simulink model "AMCLIB_FW_BAM"  (Simulink 9.3)
settings: Solver=VariableStepAuto  StartTime=0.0  StopTime=10.0  RelTol=1e-3
settings Model: Creator=nxa18952  LastModifiedBy=nxa18952
settings DataIOCC: SaveFormat=Dataset  SignalLoggingSaveFormat=Dataset  ReturnWorkspaceOutputs=on
settings OptimizationCC: LifeSpan=auto
settings DebuggingCC: UnderspecifiedInitializationDetection=Simplified  MergeDetectMultiDrivingBlocksExec=error  FcnCallInpInsideContextMsg=error  SFUnexpectedBacktrackingDiag=error  SFNoUnconditionalDefaultTransitionDiag=error  SFExecutionAtInitializationDiag=warning  ArithmeticOperatorsInVariantConditions=error
settings HardwareCC: ProdBitPerPointer=64  ProdBitPerSizeT=64  ProdBitPerPtrDiffT=64  ProdLargestAtomicFloat=Float  ProdIntDivRoundTo=Zero  ProdEndianess=LittleEndian  ProdWordSize=64  ProdHWDeviceType=Intel->x86-64 (Windows64)
settings ModelReferenceCC: PropagateSignalLabelsOutOfModel=on
settings SFSimCC: SimUseLocalCustomCode=on
settings RTWCC: RTWUseLocalCustomCode=on
settings CodeAppCC: StateflowObjectComments=off
settings GRTTargetCC: TargetLangStandard=C99 (ISO)  CombineOutputUpdateFcns=on  GRTInterface=off
settings ConfigComp: CovMetricSettings=dwe  CovHtmlReporting=off  CovSaveCumulativeToWorkspaceVar=off  CovSaveSingleToWorkspaceVar=off  CovExternalEMLEnable=on

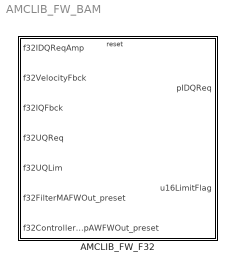
== system AMCLIB_FW_BAM ==
  AMCLIB_FW_F32 : Subsystem  TreatAsAtomicUnit=on  mask(AMCLIB_FW_F32){showStates=Hide (faster execution), resetStatesEnable=Pre-set according to the first set of inputs after reset, showDebugOutputs=Hide, u16NSamples=0, f32PropGain=0, f32IntegGain=0, s16PropGainShift=0, s16IntegGainShift=0, f32LowerLimit=0, f32UpperLimit=0}
      mask prompts: showStates "Show internal states"; resetStatesEnable "Internal state after reset"; showDebugOutputs "Show debugging outputs"; u16NSamples "u16NSamples (GDFLIB_FilterMA - recalculated smoothing factor)"; f32PropGain "f32PropGain (GFLIB_ControllerPIpAW - proportional gain)"; f32IntegGain "f32IntegGain (GFLIB_ControllerPIpAW - integral gain)"; s16PropGainShift "s16PropGainShift (GFLIB_ControllerPIpAW - scaling bitwise shift applied to the proportional gain)"; s16IntegGainShift "s16IntegGainShift (GFLIB_ControllerPIpAW - scaling bitwise shift applied to the integral gain)"; f32LowerLimit "f32LowerLimit (GFLIB_ControllerPIpAW - lower limit)"; f32UpperLimit "f32UpperLimit (GFLIB_ControllerPIpAW - upper limit)"
      mask help: Field Weakening controller for the PMSM field-oriented control algorithm in 32-bit fixed-point fractional implementation. This block supports re-initialization of the internal state during simulation. If the block is reset, the output of the MA filter and PI controller will be aligned with the inputs f32FilterMAFWOut_preset and f32ControllerPIpAWFWOut_preset. Refer to the AMMCLIB User's Guide for further details.
      mask init:
      | if ~evalin('base','exist(''tS8'',''var'')')
      |   if (2 ~= exist('SWLIBS_Typedefs.mat','file'))
      |       error('File SWLIBS_Typedefs.mat is not on the Matlab path. Please add the AMMCLIB "bam" folder in the Matlab Search Path.');
      |   else
      |       evalin('base', 'load(''SWLIBS_Typedefs.mat'')');
      |   end
      | end
      | if showStates == 1
      |     % hidden state variables
      |     if strcmp(get_param([gcb '/u16NSamples'], 'BlockType'), 'Inport')
      |         posblk = get_param(gcb, 'Position');
      | 
      |         pos = get_param(    [gcb, '/u16NSamples'], 'Position');
      |         orient = get_param( [gcb, '/u16NSamples'], 'Orientation');
      |         delete_block(       [gcb, '/u16NSamples']);
      |         add_block('built-in/Ground', [gcb, '/u16NSamples'], 'Position', pos, 'Orientation', orient);
      | 
      |         pos = get_param(    [gcb, '/f32PropGain'], 'Position');
      |         orient = get_param( [gcb, '/f32PropGain'], 'Orientation');
      |         delete_block(       [gcb, '/f32PropGain']);
      |         add_block('built-in/Ground', [gcb, '/f32PropGain'], 'Position', pos, 'Orientation', orient);
      | 
      |         pos = get_param(    [gcb, '/f32IntegGain'], 'Position');
      |         orient = get_param( [gcb, '/f32IntegGain'], 'Orientation');
      |         delete_block(       [gcb, '/f32IntegGain']);
      |         add_block('built-in/Ground', [gcb, '/f32IntegGain'], 'Position', pos, 'Orientation', orient);
      | 
      |         pos = get_param(    [gcb, '/s16PropGainShift'], 'Position');
      |         orient = get_param( [gcb, '/s16PropGainShift'], 'Orientation');
      |         delete_block(       [gcb, '/s16PropGainShift']);
      |         add_block('built-in/Ground', [gcb, '/s16PropGainShift'], 'Position', pos, 'Orientation', orient);
      | 
      |         pos = get_param(    [gcb, '/s16IntegGainShift'], 'Position');
      |         orient = get_param( [gcb, '/s16IntegGainShift'], 'Orientation');
      |         delete_block(       [gcb, '/s16IntegGainShift']);
      |         add_block('built-in/Ground', [gcb, '/s16IntegGainShift'], 'Position', pos, 'Orientation', orient);
      | 
      |         pos = get_param(    [gcb, '/f32LowerLimit'], 'Position');
      |         orient = get_param( [gcb, '/f32LowerLimit'], 'Orientation');
      |         delete_block(       [gcb, '/f32LowerLimit']);
      |         add_block('built-in/Ground', [gcb, '/f32LowerLimit'], 'Position', pos, 'Orientation', orient);
      | 
      |         pos = get_param(    [gcb, '/f32UpperLimit'], 'Position');
      |         orient = get_param( [gcb, '/f32UpperLimit'], 'Orientation');
      |         delete_block(       [gcb, '/f32UpperLimit']);
      |         add_block('built-in/Ground', [gcb, '/f32UpperLimit'], 'Position', pos, 'Orientation', orient);
      | 
      |         pos = get_param(    [gcb, '/f32IQReqK_1'], 'Position');
      |         orient = get_param( [gcb, '/f32IQReqK_1'], 'Orientation');
      |         delete_block(       [gcb, '/f32IQReqK_1']);
      |         add_block('built-in/Ground', [gcb, '/f32IQReqK_1'], 'Position', pos, 'Orientation', orient);
      | 
      |         pos = get_param(    [gcb, '/f32Acc'], 'Position');
      |         orient = get_param( [gcb, '/f32Acc'], 'Orientation');
      |         delete_block(       [gcb, '/f32Acc']);
      |         add_block('built-in/Ground', [gcb, '/f32Acc'], 'Position', pos, 'Orientation', orient);
      | 
      |         pos = get_param(    [gcb, '/f32IntegPartK_1'], 'Position');
      |         orient = get_param( [gcb, '/f32IntegPartK_1'], 'Orientation');
      |         delete_block(       [gcb, '/f32IntegPartK_1']);
      |         add_block('built-in/Ground', [gcb, '/f32IntegPartK_1'], 'Position', pos, 'Orientation', orient);
      | 
      |         pos = get_param(    [gcb, '/f32InK_1'], 'Position');
      |         orient = get_param( [gcb, '/f32InK_1'], 'Orientation');
      |         delete_block(       [gcb, '/f32InK_1']);
      |         add_block('built-in/Ground', [gcb, '/f32InK_1'], 'Position', pos, 'Orientation', orient);
      | 
      | 
      |         pos = get_param(    [gcb '/f32Acc_Out'], 'Position');
      |         orient = get_param( [gcb '/f32Acc_Out'], 'Orientation');
      |         delete_block(       [gcb '/f32Acc_Out']);
      |         add_block('built-in/Terminator', [gcb '/f32Acc_Out'], 'Position', pos, 'Orientation', orient);
      | 
      |         pos = get_param(    [gcb '/f32IntegPartK_1_Out'], 'Position');
      |         orient = get_param( [gcb '/f32IntegPartK_1_Out'], 'Orientation');
      |         delete_block(       [gcb '/f32IntegPartK_1_Out']);
      |         add_block('built-in/Terminator', [gcb '/f32IntegPartK_1_Out'], 'Position', pos, 'Orientation', orient);
      | 
      |         pos = get_param(    [gcb '/f32InK_1_Out'], 'Position');
      |         orient = get_param( [gcb '/f32InK_1_Out'], 'Orientation');
      |         delete_block(       [gcb '/f32InK_1_Out']);
      |         add_block('built-in/Terminator', [gcb '/f32InK_1_Out'], 'Position', pos, 'Orientation', orient);
      | 
      | 
      |         if strcmp(get_param([gcb '/f32IQErrSign'], 'BlockType'), 'Outport')
      |             pos = get_param(    [gcb '/f32IQErrSign'], 'Position');
      |             orient = get_param( [gcb '/f32IQErrSign'], 'Orientation');
      |             delete_block(       [gcb '/f32IQErrSign']);
      |             add_block('built-in/Terminator', [gcb '/f32IQErrSign'], 'Position', pos, 'Orientation', orient);
      | 
      |             pos = get_param(    [gcb '/f32IQErr'], 'Position');
      |             orient = get_param( [gcb '/f32IQErr'], 'Orientation');
      |             delete_block(       [gcb '/f32IQErr']);
      |             add_block('built-in/Terminator', [gcb '/f32IQErr'], 'Position', pos, 'Orientation', orient);
      | 
      |             pos = get_param(    [gcb '/f32FWErr'], 'Position');
      |             orient = get_param( [gcb '/f32FWErr'], 'Orientation');
      |             delete_block(       [gcb '/f32FWErr']);
      |             add_block('built-in/Terminator', [gcb '/f32FWErr'], 'Position', pos, 'Orientation', orient);
      | 
      |             pos = get_param(    [gcb '/f32UQErr'], 'Position');
      |             orient = get_param( [gcb '/f32UQErr'], 'Orientation');
      |             delete_block(       [gcb '/f32UQErr']);
      |             add_block('built-in/Terminator', [gcb '/f32UQErr'], 'Position', pos, 'Orientation', orient);
      | 
      |             pos = get_param(    [gcb '/f32FWErrFilt'], 'Position');
      |             orient = get_param( [gcb '/f32FWErrFilt'], 'Orientation');
      |             delete_block(       [gcb '/f32FWErrFilt']);
      |             add_block('built-in/Terminator', [gcb '/f32FWErrFilt'], 'Position', pos, 'Orientation', orient);
      | 
      |             pos = get_param(    [gcb '/f32FWAngle'], 'Position');
      |             orient = get_param( [gcb '/f32FWAngle'], 'Orientation');
      |             delete_block(       [gcb '/f32FWAngle']);
      |             add_block('built-in/Terminator', [gcb '/f32FWAngle'], 'Position', pos, 'Orientation', orient);
      | 
      |             pos = get_param(    [gcb '/f32FWSin'], 'Position');
      |             orient = get_param( [gcb '/f32FWSin'], 'Orientation');
      |             delete_block(       [gcb '/f32FWSin']);
      |             add_block('built-in/Terminator', [gcb '/f32FWSin'], 'Position', pos, 'Orientation', orient);
      | 
      |             pos = get_param(    [gcb '/f32FWCos'], 'Position');
      |             orient = get_param( [gcb '/f32FWCos'], 'Orientation');
      |             delete_block(       [gcb '/f32FWCos']);
      |             add_block('built-in/Terminator', [gcb '/f32FWCos'], 'Position', pos, 'Orientation', orient);
      | 
      |         end
      | 
      |         set_param([gcb '/f32IDQReqAmp'], 'Port', '1');
      |         set_param([gcb '/f32VelocityFbck'], 'Port', '2');
      |         set_param([gcb '/f32IQFbck'], 'Port', '3');
      |         set_param([gcb '/f32UQReq'], 'Port', '4');
      |         set_param([gcb '/f32UQLim'], 'Port', '5');
      |         set_param([gcb '/f32FilterMAFWOut_preset'], 'Port', '6');
      |         set_param([gcb '/f32ControllerPIpAWFWOut_preset'], 'Port', '7');
      | 
      |         set_param([gcb '/pIDQReq'], 'Port', '1');
      |         set_param([gcb '/u16LimitFlag'], 'Port', '2');
      | 
      |         set_param(gcb,'MaskEnables',{'on','on','off','on','on','on','on','on','on','on'});
      | 
      |         if (posblk(4) - posblk(2)) > 200
      |           height = 200;
      |           set_param(gcb,'Position',[posblk(1), posblk(2), posblk(3), posblk(2)+height])
      |         end
      |     end
      | else
      |     % shown state variables
      |     if strcmp(get_param([gcb '/u16NSamples'], 'BlockType'), 'Ground')
      |         posblk = get_param(gcb, 'Position');
      | 
      |         pos = get_param(    [gcb, '/u16NSamples'], 'Position');
      |         orient = get_param( [gcb, '/u16NSamples'], 'Orientation');
      |         delete_block(       [gcb, '/u16NSamples']);
      |         add_block('built-in/Inport', [gcb, '/u16NSamples'], 'Position', pos, 'Orientation', orient, 'OutDataTypeStr', 'uint16');
      | 
      |         pos = get_param(    [gcb, '/f32PropGain'], 'Position');
      |         orient = get_param( [gcb, '/f32PropGain'], 'Orientation');
      |         delete_block(       [gcb, '/f32PropGain']);
      |         add_block('built-in/Inport', [gcb, '/f32PropGain'], 'Position', pos, 'Orientation', orient, 'OutDataTypeStr', 'int32');
      | 
      |         pos = get_param(    [gcb, '/f32IntegGain'], 'Position');
      |         orient = get_param( [gcb, '/f32IntegGain'], 'Orientation');
      |         delete_block(       [gcb, '/f32IntegGain']);
      |         add_block('built-in/Inport', [gcb, '/f32IntegGain'], 'Position', pos, 'Orientation', orient, 'OutDataTypeStr', 'int32');
      | 
      |         pos = get_param(    [gcb, '/s16PropGainShift'], 'Position');
      |         orient = get_param( [gcb, '/s16PropGainShift'], 'Orientation');
      |         delete_block(       [gcb, '/s16PropGainShift']);
      |         add_block('built-in/Inport', [gcb, '/s16PropGainShift'], 'Position', pos, 'Orientation', orient, 'OutDataTypeStr', 'int16');
      | 
      |         pos = get_param(    [gcb, '/s16IntegGainShift'], 'Position');
      |         orient = get_param( [gcb, '/s16IntegGainShift'], 'Orientation');
      |         delete_block(       [gcb, '/s16IntegGainShift']);
      |         add_block('built-in/Inport', [gcb, '/s16IntegGainShift'], 'Position', pos, 'Orientation', orient, 'OutDataTypeStr', 'int16');
      | 
      |         pos = get_param(    [gcb, '/f32LowerLimit'], 'Position');
      |         orient = get_param( [gcb, '/f32LowerLimit'], 'Orientation');
      |         delete_block(       [gcb, '/f32LowerLimit']);
      |         add_block('built-in/Inport', [gcb, '/f32LowerLimit'], 'Position', pos, 'Orientation', orient, 'OutDataTypeStr', 'int32');
      | 
      |         pos = get_param(    [gcb, '/f32UpperLimit'], 'Position');
      |         orient = get_param( [gcb, '/f32UpperLimit'], 'Orientation');
      |         delete_block(       [gcb, '/f32UpperLimit']);
      |         add_block('built-in/Inport', [gcb, '/f32UpperLimit'], 'Position', pos, 'Orientation', orient, 'OutDataTypeStr', 'int32');
      | 
      |         pos = get_param(    [gcb, '/f32IQReqK_1'], 'Position');
      |         orient = get_param( [gcb, '/f32IQReqK_1'], 'Orientation');
      |         delete_block(       [gcb, '/f32IQReqK_1']);
      |         add_block('built-in/Inport', [gcb, '/f32IQReqK_1'], 'Position', pos, 'Orientation', orient, 'OutDataTypeStr', 'int32');
      | 
      |         pos = get_param(    [gcb, '/f32Acc'], 'Position');
      |         orient = get_param( [gcb, '/f32Acc'], 'Orientation');
      |         delete_block(       [gcb, '/f32Acc']);
      |         add_block('built-in/Inport', [gcb, '/f32Acc'], 'Position', pos, 'Orientation', orient, 'OutDataTypeStr', 'int32');
      | 
      |         pos = get_param(    [gcb, '/f32IntegPartK_1'], 'Position');
      |         orient = get_param( [gcb, '/f32IntegPartK_1'], 'Orientation');
      |         delete_block(       [gcb, '/f32IntegPartK_1']);
      |         add_block('built-in/Inport', [gcb, '/f32IntegPartK_1'], 'Position', pos, 'Orientation', orient, 'OutDataTypeStr', 'int32');
      | 
      |         pos = get_param(    [gcb, '/f32InK_1'], 'Position');
      |         orient = get_param( [gcb, '/f32InK_1'], 'Orientation');
      |         delete_block(       [gcb, '/f32InK_1']);
      |         add_block('built-in/Inport', [gcb, '/f32InK_1'], 'Position', pos, 'Orientation', orient, 'OutDataTypeStr', 'int32');
      | 
      | 
      |         pos = get_param(    [gcb '/f32Acc_Out'], 'Position');
      |         orient = get_param( [gcb '/f32Acc_Out'], 'Orientation');
      |         delete_block(       [gcb '/f32Acc_Out']);
      |         add_block('built-in/Outport', [gcb '/f32Acc_Out'], 'Position', pos, 'Orientation', orient);
      | 
      |         pos = get_param(    [gcb '/f32IntegPartK_1_Out'], 'Position');
      |         orient = get_param( [gcb '/f32IntegPartK_1_Out'], 'Orientation');
      |         delete_block(       [gcb '/f32IntegPartK_1_Out']);
      |         add_block('built-in/Outport', [gcb '/f32IntegPartK_1_Out'], 'Position', pos, 'Orientation', orient);
      | 
      |         pos = get_param(    [gcb '/f32InK_1_Out'], 'Position');
      |         orient = get_param( [gcb '/f32InK_1_Out'], 'Orientation');
      |         delete_block(       [gcb '/f32InK_1_Out']);
      |         add_block('built-in/Outport', [gcb '/f32InK_1_Out'], 'Position', pos, 'Orientation', orient);
      | 
      | 
      |         if (showDebugOutputs == 2) && (strcmp(get_param([gcb '/f32IQErrSign'], 'BlockType'), 'Terminator'))
      |             pos = get_param(    [gcb '/f32IQErrSign'], 'Position');
      |             orient = get_param( [gcb '/f32IQErrSign'], 'Orientation');
      |             delete_block(       [gcb '/f32IQErrSign']);
      |             add_block('built-in/Outport', [gcb '/f32IQErrSign'], 'Position', pos, 'Orientation', orient);
      | 
      |             pos = get_param(    [gcb '/f32IQErr'], 'Position');
      |             orient = get_param( [gcb '/f32IQErr'], 'Orientation');
      |             delete_block(       [gcb '/f32IQErr']);
      |             add_block('built-in/Outport', [gcb '/f32IQErr'], 'Position', pos, 'Orientation', orient);
      | 
      |             pos = get_param(    [gcb '/f32FWErr'], 'Position');
      |             orient = get_param( [gcb '/f32FWErr'], 'Orientation');
      |             delete_block(       [gcb '/f32FWErr']);
      |             add_block('built-in/Outport', [gcb '/f32FWErr'], 'Position', pos, 'Orientation', orient);
      | 
      |             pos = get_param(    [gcb '/f32UQErr'], 'Position');
      |             orient = get_param( [gcb '/f32UQErr'], 'Orientation');
      |             delete_block(       [gcb '/f32UQErr']);
      |             add_block('built-in/Outport', [gcb '/f32UQErr'], 'Position', pos, 'Orientation', orient);
      | 
      |             pos = get_param(    [gcb '/f32FWErrFilt'], 'Position');
      |             orient = get_param( [gcb '/f32FWErrFilt'], 'Orientation');
      |             delete_block(       [gcb '/f32FWErrFilt']);
      |             add_block('built-in/Outport', [gcb '/f32FWErrFilt'], 'Position', pos, 'Orientation', orient);
      | 
      |             pos = get_param(    [gcb '/f32FWAngle'], 'Position');
      |             orient = get_param( [gcb '/f32FWAngle'], 'Orientation');
      |             delete_block(       [gcb '/f32FWAngle']);
      |             add_block('built-in/Outport', [gcb '/f32FWAngle'], 'Position', pos, 'Orientation', orient);
      | 
      |             pos = get_param(    [gcb '/f32FWSin'], 'Position');
      |             orient = get_param( [gcb '/f32FWSin'], 'Orientation');
      |             delete_block(       [gcb '/f32FWSin']);
      |             add_block('built-in/Outport', [gcb '/f32FWSin'], 'Position', pos, 'Orientation', orient);
      | 
      |             pos = get_param(    [gcb '/f32FWCos'], 'Position');
      |             orient = get_param( [gcb '/f32FWCos'], 'Orientation');
      |             delete_block(       [gcb '/f32FWCos']);
      |             add_block('built-in/Outport', [gcb '/f32FWCos'], 'Position', pos, 'Orientation', orient);
      | 
      |         end
      | 
      |         set_param([gcb '/f32IDQReqAmp'], 'Port', '1');
      |         set_param([gcb '/f32VelocityFbck'], 'Port', '2');
      |         set_param([gcb '/f32IQFbck'], 'Port', '3');
      |         set_param([gcb '/f32UQReq'], 'Port', '4');
      |         set_param([gcb '/f32UQLim'], 'Port', '5');
      |         set_param([gcb '/f32FilterMAFWOut_preset'], 'Port', '6');
      |         set_param([gcb '/f32ControllerPIpAWFWOut_preset'], 'Port', '7');
      |         set_param([gcb '/u16NSamples'], 'Port', '8');
      |         set_param([gcb '/f32PropGain'], 'Port', '9');
      |         set_param([gcb '/f32IntegGain'], 'Port', '10');
      |         set_param([gcb '/s16PropGainShift'], 'Port', '11');
      |         set_param([gcb '/s16IntegGainShift'], 'Port', '12');
      |         set_param([gcb '/f32LowerLimit'], 'Port', '13');
      |         set_param([gcb '/f32UpperLimit'], 'Port', '14');
      |         set_param([gcb '/f32IQReqK_1'], 'Port', '15');
      |         set_param([gcb '/f32Acc'], 'Port', '16');
      |         set_param([gcb '/f32IntegPartK_1'], 'Port', '17');
      |         set_param([gcb '/f32InK_1'], 'Port', '18');
      | 
      |         if (showDebugOutputs == 2)
      |             set_param([gcb '/pIDQReq'], 'Port', '1');
      |             set_param([gcb '/u16LimitFlag'], 'Port', '2');
      |             set_param([gcb '/f32IQErrSign'], 'Port', '3');
      |             set_param([gcb '/f32IQErr'], 'Port', '4');
      |             set_param([gcb '/f32FWErr'], 'Port', '5');
      |             set_param([gcb '/f32UQErr'], 'Port', '6');
      |             set_param([gcb '/f32FWErrFilt'], 'Port', '7');
      |             set_param([gcb '/f32FWAngle'], 'Port', '8');
      |             set_param([gcb '/f32FWSin'], 'Port', '9');
      |             set_param([gcb '/f32FWCos'], 'Port', '10');
      |             set_param([gcb '/f32Acc_Out'], 'Port', '11');
      |             set_param([gcb '/f32IntegPartK_1_Out'], 'Port', '12');
      |             set_param([gcb '/f32InK_1_Out'], 'Port', '13');
      |         else
      |             set_param([gcb '/pIDQReq'], 'Port', '1');
      |             set_param([gcb '/u16LimitFlag'], 'Port', '2');
      |             set_param([gcb '/f32Acc_Out'], 'Port', '3');
      |             set_param([gcb '/f32IntegPartK_1_Out'], 'Port', '4');
      |             set_param([gcb '/f32InK_1_Out'], 'Port', '5');
      |         end
      | 
      |         set_param(gcb,'MaskEnables',{'on','on','on','off','off','off','off','off','off','off'});
      | 
      |         if (posblk(4) - posblk(2)) < 475
      |           height = 475;
      |           set_param(gcb,'Position',[posblk(1), posblk(2), posblk(3), posblk(2)+height])
      |         end
      |     else
      |         if (showDebugOutputs == 2) && (strcmp(get_param([gcb '/f32IQErrSign'], 'BlockType'), 'Terminator'))
      |             % shown debugging outputs
      |             pos = get_param(    [gcb '/f32IQErrSign'], 'Position');
      |             orient = get_param( [gcb '/f32IQErrSign'], 'Orientation');
      |             delete_block(       [gcb '/f32IQErrSign']);
      |             add_block('built-in/Outport', [gcb '/f32IQErrSign'], 'Position', pos, 'Orientation', orient);
      | 
      |             pos = get_param(    [gcb '/f32IQErr'], 'Position');
      |             orient = get_param( [gcb '/f32IQErr'], 'Orientation');
      |             delete_block(       [gcb '/f32IQErr']);
      |             add_block('built-in/Outport', [gcb '/f32IQErr'], 'Position', pos, 'Orientation', orient);
      | 
      |             pos = get_param(    [gcb '/f32FWErr'], 'Position');
      |             orient = get_param( [gcb '/f32FWErr'], 'Orientation');
      |             delete_block(       [gcb '/f32FWErr']);
      |             add_block('built-in/Outport', [gcb '/f32FWErr'], 'Position', pos, 'Orientation', orient);
      | 
      |             pos = get_param(    [gcb '/f32UQErr'], 'Position');
      |             orient = get_param( [gcb '/f32UQErr'], 'Orientation');
      |             delete_block(       [gcb '/f32UQErr']);
      |             add_block('built-in/Outport', [gcb '/f32UQErr'], 'Position', pos, 'Orientation', orient);
      | 
      |             pos = get_param(    [gcb '/f32FWErrFilt'], 'Position');
      |             orient = get_param( [gcb '/f32FWErrFilt'], 'Orientation');
      |             delete_block(       [gcb '/f32FWErrFilt']);
      |             add_block('built-in/Outport', [gcb '/f32FWErrFilt'], 'Position', pos, 'Orientation', orient);
      | 
      |             pos = get_param(    [gcb '/f32FWAngle'], 'Position');
      |             orient = get_param( [gcb '/f32FWAngle'], 'Orientation');
      |             delete_block(       [gcb '/f32FWAngle']);
      |             add_block('built-in/Outport', [gcb '/f32FWAngle'], 'Position', pos, 'Orientation', orient);
      | 
      |             pos = get_param(    [gcb '/f32FWSin'], 'Position');
      |             orient = get_param( [gcb '/f32FWSin'], 'Orientation');
      |             delete_block(       [gcb '/f32FWSin']);
      |             add_block('built-in/Outport', [gcb '/f32FWSin'], 'Position', pos, 'Orientation', orient);
      | 
      |             pos = get_param(    [gcb '/f32FWCos'], 'Position');
      |             orient = get_param( [gcb '/f32FWCos'], 'Orientation');
      |             delete_block(       [gcb '/f32FWCos']);
      |             add_block('built-in/Outport', [gcb '/f32FWCos'], 'Position', pos, 'Orientation', orient);
      | 
      |             set_param([gcb '/pIDQReq'], 'Port', '1');
      |             set_param([gcb '/u16LimitFlag'], 'Port', '2');
      |             set_param([gcb '/f32IQErrSign'], 'Port', '3');
      |             set_param([gcb '/f32IQErr'], 'Port', '4');
      |             set_param([gcb '/f32FWErr'], 'Port', '5');
      |             set_param([gcb '/f32UQErr'], 'Port', '6');
      |             set_param([gcb '/f32FWErrFilt'], 'Port', '7');
      |             set_param([gcb '/f32FWAngle'], 'Port', '8');
      |             set_param([gcb '/f32FWSin'], 'Port', '9');
      |             set_param([gcb '/f32FWCos'], 'Port', '10');
      |             set_param([gcb '/f32Acc_Out'], 'Port', '11');
      |             set_param([gcb '/f32IntegPartK_1_Out'], 'Port', '12');
      |             set_param([gcb '/f32InK_1_Out'], 'Port', '13');
      |         elseif (showDebugOutputs == 1) && (strcmp(get_param([gcb '/f32IQErrSign'], 'BlockType'), 'Outport'))
      |             % hidden debugging outputs
      |             pos = get_param(    [gcb '/f32IQErrSign'], 'Position');
      |             orient = get_param( [gcb '/f32IQErrSign'], 'Orientation');
      |             delete_block(       [gcb '/f32IQErrSign']);
      |             add_block('built-in/Terminator', [gcb '/f32IQErrSign'], 'Position', pos, 'Orientation', orient);
      | 
      |             pos = get_param(    [gcb '/f32IQErr'], 'Position');
      |             orient = get_param( [gcb '/f32IQErr'], 'Orientation');
      |             delete_block(       [gcb '/f32IQErr']);
      |             add_block('built-in/Terminator', [gcb '/f32IQErr'], 'Position', pos, 'Orientation', orient);
      | 
      |             pos = get_param(    [gcb '/f32FWErr'], 'Position');
      |             orient = get_param( [gcb '/f32FWErr'], 'Orientation');
      |             delete_block(       [gcb '/f32FWErr']);
      |             add_block('built-in/Terminator', [gcb '/f32FWErr'], 'Position', pos, 'Orientation', orient);
      | 
      |             pos = get_param(    [gcb '/f32UQErr'], 'Position');
      |             orient = get_param( [gcb '/f32UQErr'], 'Orientation');
      |             delete_block(       [gcb '/f32UQErr']);
      |             add_block('built-in/Terminator', [gcb '/f32UQErr'], 'Position', pos, 'Orientation', orient);
      | 
      |             pos = get_param(    [gcb '/f32FWErrFilt'], 'Position');
      |             orient = get_param( [gcb '/f32FWErrFilt'], 'Orientation');
      |             delete_block(       [gcb '/f32FWErrFilt']);
      |             add_block('built-in/Terminator', [gcb '/f32FWErrFilt'], 'Position', pos, 'Orientation', orient);
      | 
      |             pos = get_param(    [gcb '/f32FWAngle'], 'Position');
      |             orient = get_param( [gcb '/f32FWAngle'], 'Orientation');
      |             delete_block(       [gcb '/f32FWAngle']);
      |             add_block('built-in/Terminator', [gcb '/f32FWAngle'], 'Position', pos, 'Orientation', orient);
      | 
      |             pos = get_param(    [gcb '/f32FWSin'], 'Position');
      |             orient = get_param( [gcb '/f32FWSin'], 'Orientation');
      |             delete_block(       [gcb '/f32FWSin']);
      |             add_block('built-in/Terminator', [gcb '/f32FWSin'], 'Position', pos, 'Orientation', orient);
      | 
      |             pos = get_param(    [gcb '/f32FWCos'], 'Position');
      |             orient = get_param( [gcb '/f32FWCos'], 'Orientation');
      |             delete_block(       [gcb '/f32FWCos']);
      |             add_block('built-in/Terminator', [gcb '/f32FWCos'], 'Position', pos, 'Orientation', orient);
      | 
      |             set_param([gcb '/pIDQReq'], 'Port', '1');
      |             set_param([gcb '/u16LimitFlag'], 'Port', '2');
      |             set_param([gcb '/f32Acc_Out'], 'Port', '3');
      |             set_param([gcb '/f32IntegPartK_1_Out'], 'Port', '4');
      |             set_param([gcb '/f32InK_1_Out'], 'Port', '5');
      |         end
      |     end
      | end
      settings: RTWSystemCode=Inline
      mask TypeOptions showStates: Hide (faster execution) | Show (allows debugging; connect feedback loops manually)
      mask Callback showStates:
      | maskStr = get_param(gcb,'showStates');
      | if strcmp(maskStr,'Hide (faster execution)'),
      |     set_param(gcb,'MaskEnables',{'on','on','off','on','on','on','on','on','on','on'});
      | else
      |     set_param(gcb,'MaskEnables',{'on','on','on','off','off','off','off','off','off','off'});
      | end
      mask TypeOptions resetStatesEnable: Pre-set according to the first set of inputs after reset | Clear to zero
      mask TypeOptions showDebugOutputs: Hide | Show
      mask Display:
      | color('black');
      | pos = get_param(gcb, 'Position');
      | width = pos(3) - pos(1);
      | height = pos(4) - pos(2);
      | tX=width/2;
      | tY=height - 25;
      | color('black');
      | text(tX,tY, 'AMCLIB_FW_F32', 'horizontalAlignment', 'center');
      | if showStates == 2
      |   color('red');
      |   text(tX,tY - 20, ['debugging mode' char(13) char(10) '(limited performance)'], 'horizontalAlignment', 'center');
      | end

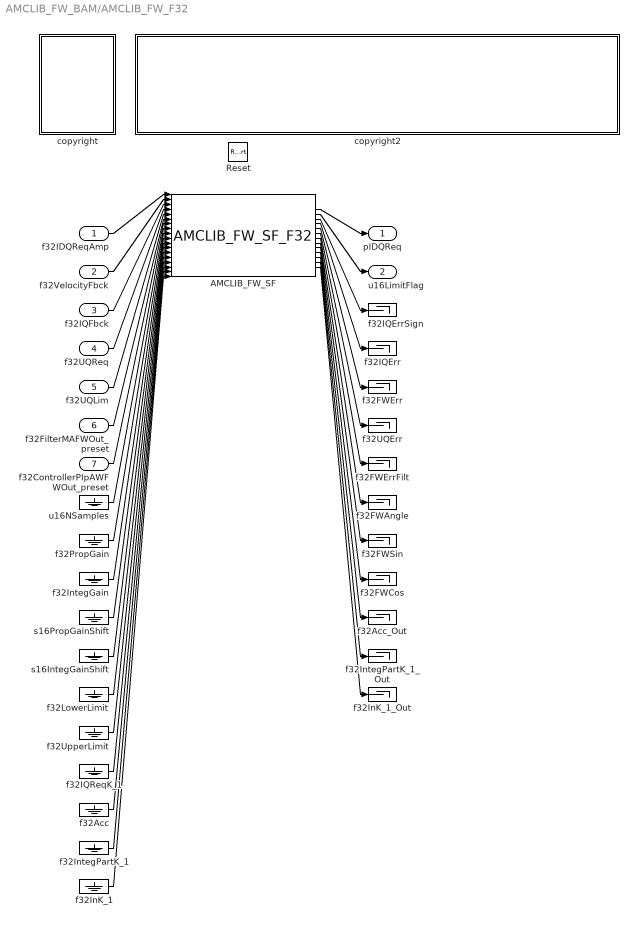
== system AMCLIB_FW_BAM/AMCLIB_FW_F32 ==
  f32IDQReqAmp : Inport  OutDataTypeStr=int32
  f32VelocityFbck : Inport  Port=2  OutDataTypeStr=int32
  f32IQFbck : Inport  Port=3  OutDataTypeStr=int32
  f32UQReq : Inport  Port=4  OutDataTypeStr=int32
  f32UQLim : Inport  Port=5  OutDataTypeStr=int32
  f32FilterMAFWOut_preset : Inport  Port=6  OutDataTypeStr=int32
  f32ControllerPIpAWFWOut_preset : Inport  Port=7  OutDataTypeStr=int32
  Reset : ResetPort  DisableCoverage=on
  AMCLIB_FW_SF : S-Function  FunctionName=AMCLIB_FW_SF_F32  Parameters=showStates,resetStatesEnable,showDebugOutputs,u16NSamples,f32PropGain,f32IntegGain,s16PropGainShift,s16IntegGainShift,f32LowerLimit,f32UpperLimit  SFunctionDeploymentMode=off  EnableBusSupport=off
  copyright : Subsystem
      mask Display: text(10,90,'FILE:');text(10,75,'DESRIPTION:');text(10,60,'COPYRIGHT:');text(10,45,'VERSION:');text(10,30,'DATE:')
  copyright2 : Subsystem
      mask Display: text(10,90,'AMCLIB_FW_BAM_F32.mdl');text(10,75,'PMSM Field Weakening Controller');text(10,60,'NXP 2020');text(10,45,'1.0');text(10,30,'28-Mar-2020');
  f32Acc : Ground
  f32Acc_Out : Terminator
  f32FWAngle : Terminator
  f32FWCos : Terminator
  f32FWErr : Terminator
  f32FWErrFilt : Terminator
  f32FWSin : Terminator
  f32IQErr : Terminator
  f32IQErrSign : Terminator
  f32IQReqK_1 : Ground
  f32InK_1 : Ground
  f32InK_1_Out : Terminator
  f32IntegGain : Ground
  f32IntegPartK_1 : Ground
  f32IntegPartK_1_Out : Terminator
  f32LowerLimit : Ground
  f32PropGain : Ground
  f32UQErr : Terminator
  f32UpperLimit : Ground
  s16IntegGainShift : Ground
  s16PropGainShift : Ground
  u16NSamples : Ground
  pIDQReq : Outport
  u16LimitFlag : Outport  Port=2
  wires:
  f32IDQReqAmp/1 -> AMCLIB_FW_SF/1
  f32VelocityFbck/1 -> AMCLIB_FW_SF/2
  f32IQFbck/1 -> AMCLIB_FW_SF/3
  f32UQReq/1 -> AMCLIB_FW_SF/4
  f32UQLim/1 -> AMCLIB_FW_SF/5
  f32FilterMAFWOut_preset/1 -> AMCLIB_FW_SF/6
  f32ControllerPIpAWFWOut_preset/1 -> AMCLIB_FW_SF/7
  u16NSamples/1 -> AMCLIB_FW_SF/8
  f32PropGain/1 -> AMCLIB_FW_SF/9
  f32IntegGain/1 -> AMCLIB_FW_SF/10
  s16PropGainShift/1 -> AMCLIB_FW_SF/11
  s16IntegGainShift/1 -> AMCLIB_FW_SF/12
  f32LowerLimit/1 -> AMCLIB_FW_SF/13
  f32UpperLimit/1 -> AMCLIB_FW_SF/14
  f32IQReqK_1/1 -> AMCLIB_FW_SF/15
  f32Acc/1 -> AMCLIB_FW_SF/16
  f32IntegPartK_1/1 -> AMCLIB_FW_SF/17
  f32InK_1/1 -> AMCLIB_FW_SF/18
  AMCLIB_FW_SF/1 -> pIDQReq/1
  AMCLIB_FW_SF/2 -> u16LimitFlag/1
  AMCLIB_FW_SF/3 -> f32IQErrSign/1
  AMCLIB_FW_SF/4 -> f32IQErr/1
  AMCLIB_FW_SF/5 -> f32FWErr/1
  AMCLIB_FW_SF/6 -> f32UQErr/1
  AMCLIB_FW_SF/7 -> f32FWErrFilt/1
  AMCLIB_FW_SF/8 -> f32FWAngle/1
  AMCLIB_FW_SF/9 -> f32FWSin/1
  AMCLIB_FW_SF/10 -> f32FWCos/1
  AMCLIB_FW_SF/11 -> f32Acc_Out/1
  AMCLIB_FW_SF/12 -> f32IntegPartK_1_Out/1
  AMCLIB_FW_SF/13 -> f32InK_1_Out/1

== system AMCLIB_FW_BAM/AMCLIB_FW_F32/copyright ==

== system AMCLIB_FW_BAM/AMCLIB_FW_F32/copyright2 ==
